simulink model "MRACDireto_Trab1_Regra_MIT_Pedro"  (R2015a)
settings: Solver=ode45  StartTime=0.0  StopTime=5000  FixedStep=10^-2  RelTol=1e-3
values from neighbouring files (symbols this model uses):
  b = [0 10]    [aprendizado_gamma.m]    (also in aprendizado_gamma_ini.m = [0 11])
  gamma = calc_gamma_0(K, ref, min(it), max(it), theta_estrela)    [aprendizado_gamma.m]    (also in aprendizado_gamma_ini.m)
  it = [10 1]    [aprendizado_gamma.m]    (also in aprendizado_gamma_ini.m)
  ref = 100    [aprendizado_gamma.m]    (also in aprendizado_gamma_ini.m)
  theta_c_ini = 0*(-theta_estrela+modelo_ref)    [aprendizado_gamma.m]    (also in aprendizado_gamma_ini.m = 0.7*([0 1.4205 -0.25 -5.625/11]))
settings Model: Creator=user  LastModifiedBy=user
settings SolverCC: ShapePreserveControl=EnableAll

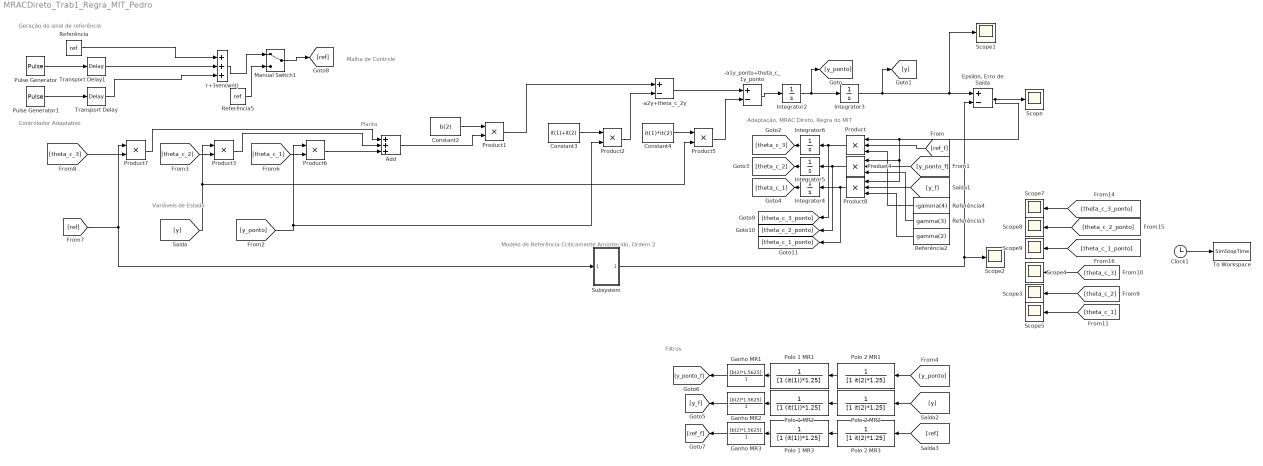
== system MRACDireto_Trab1_Regra_MIT_Pedro ==
  note: Variáveis de Estado
  note: Geração do sinal de referência
  note: Filtros
  note: Planta
  note: Malha de Controle
  note: Modelo de Referência Criticamente Amortecido, Ordem 2
  note: Controlador Adaptativo
  note: Adaptação, MRAC Direto, Regra do MIT
  "  Referência" : Constant  Value=ref
  "  Referência2" : Constant  Value=gamma(2)
  "  Referência3" : Constant  Value=gamma(3)
  "  Referência4" : Constant  Value=-gamma(4)
  "  Referência5" : Constant  Value=ref
  -a1y_ponto+theta_c_1y_ponto : Sum  Inputs=+-
  -a2y+theta_c_2y : Sum  Inputs=+-
  Add : Sum  Inputs=+++
  Clock1 : Clock
  Constant2 : Constant  Value=b(2)
  Constant3 : Constant  Value=it(1)+it(2)
  Constant4 : Constant  Value=it(1)*it(2)
  "Epsilon, Erro de Saída" : Sum  Inputs=+-
  Ganho MR1 : TransferFcn  Numerator=[b(2)*1.5625]  Denominator=[1]
  Ganho MR2 : TransferFcn  Numerator=[b(2)*1.5625]  Denominator=[1]
  Ganho MR3 : TransferFcn  Numerator=[b(2)*1.5625]  Denominator=[1]
  Integrator2 : Integrator
  Integrator3 : Integrator
  Integrator4 : Integrator  InitialCondition=theta_c_ini(4)
  Integrator5 : Integrator  InitialCondition=theta_c_ini(3)
  Integrator6 : Integrator  InitialCondition=theta_c_ini(2)
  Manual Switch1 : ManualSwitch
  Polo 1 MR1 : TransferFcn  Denominator=[1 (it(1))*1.25]
  Polo 1 MR2 : TransferFcn  Denominator=[1 (it(1))*1.25]
  Polo 1 MR3 : TransferFcn  Denominator=[1 (it(1))*1.25]
  Polo 2 MR1 : TransferFcn  Denominator=[1 it(2)*1.25]
  Polo 2 MR2 : TransferFcn  Denominator=[1 it(2)*1.25]
  Polo 2 MR3 : TransferFcn  Denominator=[1 it(2)*1.25]
  Product : Product  Inputs=3
  Product{1..3,5..7} (6 alike) : Product
  Product4 : Product  Inputs=3
  Product8 : Product  Inputs=3
  Pulse Generator : DiscretePulseGenerator  PulseType=Time based  Amplitude=ref/4  Period=0.5/sqrt(it(1)*it(2))  PulseWidth=50
  Pulse Generator1 : DiscretePulseGenerator  PulseType=Time based  Amplitude=ref/4  Period=2/sqrt(it(1)*it(2))  PulseWidth=50
  Scope{,1..5,7..9} (9 alike) : Scope
      Scope settings: TimeRange=200  YMin=-0.0275  YMax=0.025
      Scope1 settings: YMin=110  YMax=110
      Scope2 settings: YMin=123  YMax=126.5  SaveName=ScopeData2
      Scope3 settings: YMin=-0.52874  YMax=-0.52869  SaveName=ScopeData3
      Scope4 settings: YMin=1.5817  YMax=1.58177  SaveName=ScopeData4
      Scope5 settings: TimeRange=5000  YMin=-0.249135  YMax=-0.249113  SaveName=ScopeData5
      Scope7 settings: YMin=-0.0025  YMax=0.0025  SaveName=ScopeData7
      Scope8 settings: YMin=-0.0001  YMax=0.0001  SaveName=ScopeData8
      Scope9 settings: YMin=95  YMax=105  SaveName=ScopeData9
  Subsystem : Subsystem
  To Workspace : ToWorkspace  VariableName=SimStopTime  SaveFormat=Timeseries  SampleTime=-1
  Transport Delay : TransportDelay  DelayTime=100
  Transport Delay1 : TransportDelay  DelayTime=100
  r+3sen(wnt) : Sum  Inputs=+++
  wires:
  Integrator3/1 -> [y], Scope1/1, "Epsilon, Erro de Saída"/1
  Integrator2/1 -> [y_ponto], Integrator3/1
  -a1y_ponto+theta_c_1y_ponto/1 -> Integrator2/1
  -a2y+theta_c_2y/1 -> -a1y_ponto+theta_c_1y_ponto/1
  Product2/1 -> -a2y+theta_c_2y/2
  Constant3/1 -> Product2/1
  Product1/1 -> -a2y+theta_c_2y/1
  [y] -> Product5/2, Product3/1
  [theta_c_2] -> Product3/2
  Constant4/1 -> Product5/1
  [y_ponto] -> Product2/2, Product6/1
  [theta_c_1] -> Product6/2
  Product5/1 -> -a1y_ponto+theta_c_1y_ponto/2
  Constant2/1 -> Product1/1
  [theta_c_3] -> Product7/2
  [ref_f] -> Product/2
  [y_ponto_f] -> Product4/2
  [y_f] -> Product8/2
  "  Referência4"/1 -> Product/3
  "  Referência3"/1 -> Product4/3
  "  Referência2"/1 -> Product8/3
  Polo 2 MR1/1 -> Polo 1 MR1/1
  Polo 1 MR1/1 -> Ganho MR1/1
  [y_ponto] -> Polo 2 MR1/1
  Polo 2 MR2/1 -> Polo 1 MR2/1
  Polo 1 MR2/1 -> Ganho MR2/1
  [y] -> Polo 2 MR2/1
  Ganho MR1/1 -> [y_ponto_f]
  Ganho MR2/1 -> [y_f]
  Polo 2 MR3/1 -> Polo 1 MR3/1
  Polo 1 MR3/1 -> Ganho MR3/1
  [ref] -> Polo 2 MR3/1
  Ganho MR3/1 -> [ref_f]
  Integrator4/1 -> [theta_c_1]
  Product/1 -> [theta_c_3_ponto], Integrator6/1
  Integrator6/1 -> [theta_c_3]
  Product4/1 -> [theta_c_2_ponto], Integrator5/1
  Integrator5/1 -> [theta_c_2]
  [ref] -> Subsystem/1(Ref), Product7/1
  "  Referência"/1 -> r+3sen(wnt)/1
  [theta_c_2] -> Scope3/1
  [theta_c_3] -> Scope4/1
  [theta_c_1] -> Scope5/1
  Product8/1 -> [theta_c_1_ponto], Integrator4/1
  "Epsilon, Erro de Saída"/1 -> Scope/1, Product8/1, Product4/1, Product/1
  [theta_c_3_ponto] -> Scope7/1
  [theta_c_2_ponto] -> Scope8/1
  [theta_c_1_ponto] -> Scope9/1
  Manual Switch1/1 -> [ref]
  r+3sen(wnt)/1 -> Manual Switch1/1
  "  Referência5"/1 -> Manual Switch1/2
  Clock1/1 -> To Workspace/1
  Product7/1 -> Add/1
  Product3/1 -> Add/2
  Product6/1 -> Add/3
  Add/1 -> Product1/2
  Pulse Generator1/1 -> Transport Delay/1
  Pulse Generator/1 -> Transport Delay1/1
  Transport Delay1/1 -> r+3sen(wnt)/2
  Transport Delay/1 -> r+3sen(wnt)/3
  Subsystem/1(Ym) -> Scope2/1, "Epsilon, Erro de Saída"/2

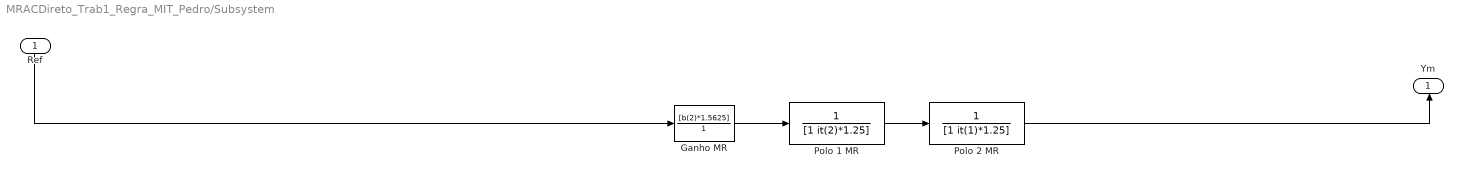
== system MRACDireto_Trab1_Regra_MIT_Pedro/Subsystem ==
  Ref : Inport
  Ganho MR : TransferFcn  Numerator=[b(2)*1.5625]  Denominator=[1]
  Polo 1 MR : TransferFcn  Denominator=[1 it(2)*1.25]
  Polo 2 MR : TransferFcn  Denominator=[1 it(1)*1.25]
  Ym : Outport
  wires:
  Polo 1 MR/1 -> Polo 2 MR/1
  Polo 2 MR/1 -> Ym/1
  Ganho MR/1 -> Polo 1 MR/1
  Ref/1 -> Ganho MR/1
